simulink model "VehicleSimulationErrorTest"  (R2018b)
settings: Solver=FixedStepAuto  StartTime=0.0  StopTime=NsimMax*Ts  FixedStep=Ts  RelTol=1e-6
values from neighbouring files (symbols this model uses):
  state0 = x0(:,i)    [errorAnalysis.m]
  Ts = 0.01    [modelFitEDMD.m]
settings Model: Creator=Marko  LastModifiedBy=Marko

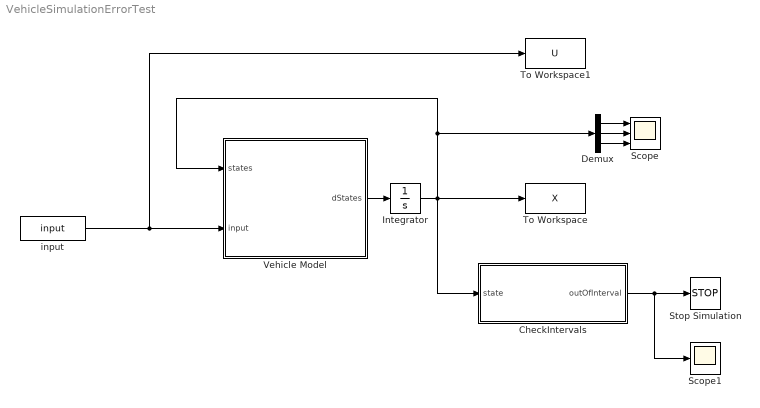
== system VehicleSimulationErrorTest ==
  CheckIntervals : MATLAB Function  TreatAsAtomicUnit=on
  Demux : Demux  Outputs=3
  Integrator : Integrator  InitialCondition=state0
  Scope : Scope  NumInputPorts=3
  Scope1 : Scope
  Stop Simulation : Stop
  To Workspace : ToWorkspace  VariableName=X  SampleTime=Ts
  To Workspace1 : ToWorkspace  VariableName=U  SampleTime=Ts
  Vehicle Model : MATLAB Function  TreatAsAtomicUnit=on
  input : FromWorkspace  VariableName=input  SampleTime=Ts
  wires:
  Vehicle Model/1(dStates) -> Integrator/1
  Integrator/1 -> CheckIntervals/1(state), To Workspace/1, Demux/1, Vehicle Model/1(states)
  Demux/1 -> Scope/1
  Demux/2 -> Scope/2
  Demux/3 -> Scope/3
  input/1 -> To Workspace1/1, Vehicle Model/2(input)
  CheckIntervals/1(outOfInterval) -> Scope1/1, Stop Simulation/1

== matlab function VehicleSimulationErrorTest/CheckIntervals ==
  data: state input; outOfInterval output
function outOfInterval = CheckIntervals(state)

vx = state(1);
vy = state(2);
omega = state(3);

inVx = vx >= 10 && vx <= 50;
inVy = vy >= -30 && vy <= 30;
inOmega = omega >= -10 && omega <= 10;

outOfInterval = ~(inVx && inVy && inOmega);

== matlab function VehicleSimulationErrorTest/Vehicle Model ==
  data: states input; dStates output; input input
function dStates = VehicleModel(states, input)
% VEHICLE MODEL 
%   The function accepts current system states and inputs, and calculates 
%   state derivatives.

% State definition
vx = states(1);
vy = states(2);
omega = states(3);

% Input definition
Fxfl = input(1);
Fyfl = input(2);
Fxfr = input(3);
Fyfr = input(4);
Fxrl = input(5);
Fxrr = input(6);

% Initialize vehicle parameters
vehicle = LoadVehicleParameters();

% Vehicle parameters
lf = vehicle.lf;
lr = vehicle.lr;
w = vehicle.w;
m = vehicle.m;
Jz = vehicle.Jz;

% Air drag parameters
cw = vehicle.cw;
rho = vehicle.rho;
Aw = vehicle.Aw;

% VEHICLE VELOCITIES

% Lateral velocities
vyrl = vy - lr*omega;
vyrr = vy - lr*omega;
% Longitudinal velocities
vxrl = vx - w*omega;
vxrr = vx + w*omega;

% TIRE VELOCITIES

% Cornering velocities
vcrl = vyrl;
vcrr = vyrr;

% Longitudinal velocities
vlrl = vxrl;
vlrr = vxrr;

% TIRE SLIP ANGLES

alpha_rl = atan2(vcrl,vlrl);
alpha_rr = atan2(vcrr,vlrr);

% TIRE FORCES
Cy = vehicle.Cy;

% Conrnering forces
Fcrl = -Cy*alpha_rl;
Fcrr = -Cy*alpha_rr;

% AXLE FORCES

% Lateral forces
Fyrl = Fcrl;
Fyrr = Fcrr;

% VEHICLE DYNAMICS MODEL

dvx = vy*omega + 1/m *(-0.5*cw*rho*Aw*sqrt(vx^2+vy^2)*vx + Fxfl + Fxfr + Fxrl + Fxrr);
dvy = -vx*omega + 1/m *(-0.5*cw*rho*Aw*sqrt(vx^2+vy^2)*vy + Fyfl + Fyfr + Fyrl + Fyrr);
dOmega = lf/Jz*(Fyfl + Fyfr) - lr/Jz*(Fyrl + Fyrr) + w/Jz*(-Fxfl + Fxfr -Fxrl + Fxrr);

dStates = [dvx; dvy; dOmega];
end
